simulink model "lunchline_ex5"  (R2016a)
settings: Solver=VariableStepAuto  StartTime=0.0  StopTime=90  RelTol=1e-3
undefined symbols (not defined in the file): m, n
settings Model: Creator=ningd  LastModifiedBy=ningd

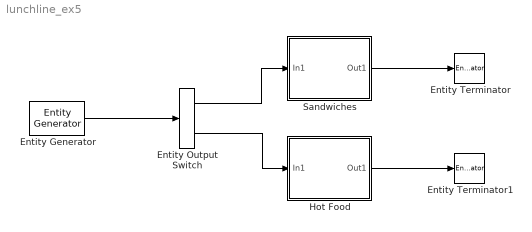
== system lunchline_ex5 ==
  Entity Output Switch : EntityOutputSwitch  InputPortMessageModes=m  OutputPortMessageModes=m,m  SwitchingCriterion=From attribute  SwitchAttributeName=Lunch
  Entity Generator : EntityGenerator  OutputPortMessageModes=m  TimeSource=MATLAB action  IntergenerationTimeAction=dt = exprnd(0.5);  GenerateEntityAtSimulationStart=off  GenerateAction=|  AttributeName=ServiceTime|Lunch  AttributeInitialValue=1|1  EntityType=Structured  EntityTypeName=Customer
      | % Define a service time from a normal distribution 
      | % with mean 1.7 and std deviation 0.2
      | entity.ServiceTime = 1.7 + 0.2*randn;
      | 
      | % Define lunch attribute as an equiprobable value 
      | % value of 1 or 2
      | entity.Lunch = randi([1,2]);
  Entity Terminator : EntityTerminator  InputPortMessageModes=m
  Entity Terminator1 : EntityTerminator  InputPortMessageModes=m
  Hot Food : Subsystem
  Sandwiches : Subsystem
  wires:
  Entity Generator/1 -> Entity Output Switch/1
  Entity Output Switch/1 -> Sandwiches/1(In1)
  Sandwiches/1(Out1) -> Entity Terminator/1
  Entity Output Switch/2 -> Hot Food/1(In1)
  Hot Food/1(Out1) -> Entity Terminator1/1

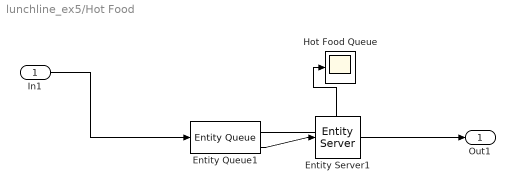
== system lunchline_ex5/Hot Food ==
  In1 : Inport
  Entity Queue1 : EntityQueue  InputPortMessageModes=m  OutputPortMessageModes=n,m  NumberEntitiesInBlock=on
      settings: OutputPortMap=o1,o5
  Entity Server1 : EntityServer  InputPortMessageModes=m  OutputPortMessageModes=m  Capacity=2  ServiceTimeSource=Attribute
  Hot Food Queue : Scope
  Out1 : Outport
  wires:
  Entity Queue1/2 -> Entity Server1/1
  Entity Server1/1 -> Out1/1
  Entity Queue1/1 -> Hot Food Queue/1
  In1/1 -> Entity Queue1/1

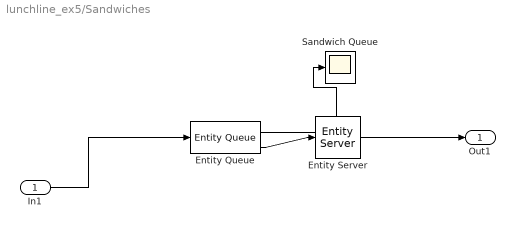
== system lunchline_ex5/Sandwiches ==
  In1 : Inport
  Entity Queue : EntityQueue  InputPortMessageModes=m  OutputPortMessageModes=n,m  NumberEntitiesInBlock=on
      settings: OutputPortMap=o1,o5
  Entity Server : EntityServer  InputPortMessageModes=m  OutputPortMessageModes=m  Capacity=2  ServiceTimeSource=Attribute
  Sandwich Queue : Scope
  Out1 : Outport
  wires:
  Entity Queue/2 -> Entity Server/1
  Entity Server/1 -> Out1/1
  Entity Queue/1 -> Sandwich Queue/1
  In1/1 -> Entity Queue/1
